simulink model "MPC_test"  (R2017a)
settings: Solver=VariableStepAuto  StartTime=0.0  StopTime=0.2  FixedStep=1e-6  RelTol=1e-3
undefined symbols (not defined in the file or in its folder): sis
libraries: mpclib x1
settings Model: Creator=erich  LastModifiedBy=erich

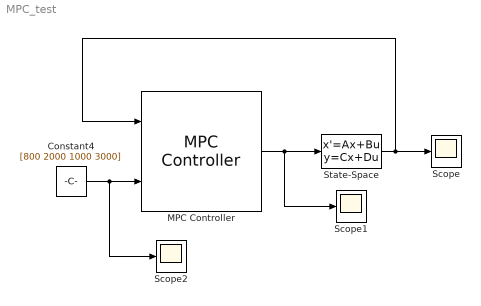
== system MPC_test ==
  Constant4 : Constant  Value=[800 2000 1000 3000]
  MPC Controller : mpclib/MPC Controller  SCDEnableBlockLinearizationSpecification=on  mpcobj=mpcobj  is_multiple=0  enable_value=0  return_u0=off  ref_from_ws=off  ref_signal_name=[]  ref_preview=off  md_from_ws=off  md_signal_name=[]  md_preview=off  from_project=off  project_file=MPCtask.mat  md_inport=off  mv_inport=off  cost_outport=off  return_sequence=off  return_qpstatus=off  return_state=off  state_inport=off  lims_inport=off  ywt_inport=off  is_designfromscratch=0  uwt_inport=off  duwt_inport=off  rhoeps_inport=off  uref_inport=off  n_ts=0.001  n_mv=4  n_md=0  n_ud=0  n_mo=4  n_uo=0  BlockDataType=double  SampleTimeInherited=off  switch_inport=off
  Scope : Scope
  Scope1 : Scope
  Scope2 : Scope
  State-Space : StateSpace  A=sis.A  B=sis.B  C=sis.C  D=sis.D  X0=0
  wires:
  MPC Controller/1 -> Scope1/1, State-Space/1
  Constant4/1 -> Scope2/1, MPC Controller/2
  State-Space/1 -> Scope/1, MPC Controller/1
